simulink model "Standard_H_Infinity_Full_Order_Synthesis"  (R2024a)
settings: Solver=VariableStepAuto  StartTime=0.0  StopTime=10.0  RelTol=1e-3
values from neighbouring files (symbols this model uses):
  Gain_Infinity_Filter_1 = 0.5    [Controller_Stochastic_Optimization.m]    (also in Standard_H_Infinity_Controller_Tuning.m)
  Gain_Infinity_Filter_2 = 100    [Controller_Stochastic_Optimization.m]    (also in Standard_H_Infinity_Controller_Tuning.m = 10000)
  Gain_Infinity_Filter_3 = 10^(Optimal_Vector(5))    [Controller_Stochastic_Optimization.m]    (also in Cost_Function_Optimal_Tuning_Controller.m; Standard_H_Infinity_Controller_Tuning.m = 10)
  Gain_Static_Filter_1 = 1000    [Controller_Stochastic_Optimization.m]    (also in Standard_H_Infinity_Controller_Tuning.m = 100)
  Gain_Static_Filter_2 = 0.01    [Controller_Stochastic_Optimization.m]    (also in Standard_H_Infinity_Controller_Tuning.m)
  Gain_Static_Filter_3 = 10^(Optimal_Vector(4))    [Controller_Stochastic_Optimization.m]    (also in Cost_Function_Optimal_Tuning_Controller.m; Standard_H_Infinity_Controller_Tuning.m = 0.1)
  Gain_Static_Filter_4 = 10^(Optimal_Vector(6))    [Controller_Stochastic_Optimization.m]    (also in Cost_Function_Optimal_Tuning_Controller.m; Standard_H_Infinity_Controller_Tuning.m = 0.1)
  Input_Matrix_Nominal_Global = [Input_Matrix_Nominal Perturbation_Input_Matrix_Nominal]    [Controller_Stochastic_Optimization.m]    (also in Standard_H_Infinity_Controller_Tuning.m)
  Input_Measurement_Matrix_Global_Nominal = [0 0]    [Controller_Stochastic_Optimization.m]    (also in Standard_H_Infinity_Controller_Tuning.m)
  Measurement_Matrix_Ship_Wave_Nominal = [0 1 1 0]    [Controller_Stochastic_Optimization.m]    (also in Standard_H_Infinity_Controller_Tuning.m)
  Pulsation_Unit_Gain_Filter_1 = 10^(Optimal_Vector(1))    [Controller_Stochastic_Optimization.m]    (also in Cost_Function_Optimal_Tuning_Controller.m; Standard_H_Infinity_Controller_Tuning.m = 0.15)
  Pulsation_Unit_Gain_Filter_2 = 10^(Optimal_Vector(2))    [Controller_Stochastic_Optimization.m]    (also in Cost_Function_Optimal_Tuning_Controller.m; Standard_H_Infinity_Controller_Tuning.m = 0.8)
  Pulsation_Unit_Gain_Filter_3 = 10^(Optimal_Vector(3))    [Controller_Stochastic_Optimization.m]    (also in Cost_Function_Optimal_Tuning_Controller.m; Standard_H_Infinity_Controller_Tuning.m = 70)
  State_Matrix_Ship_Wave_Nominal = [0 1 0 0 ... (first row only)    [Controller_Stochastic_Optimization.m]    (also in Standard_H_Infinity_Controller_Tuning.m)
settings Model: Creator=gerar  LastModifiedBy=gerar

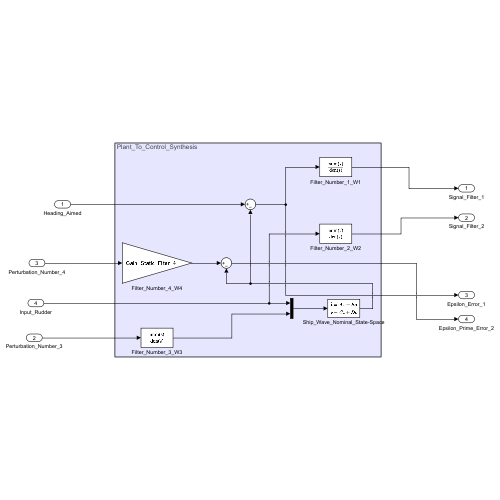
[thumbnail: Simulink's stored preview of the top-level diagram]
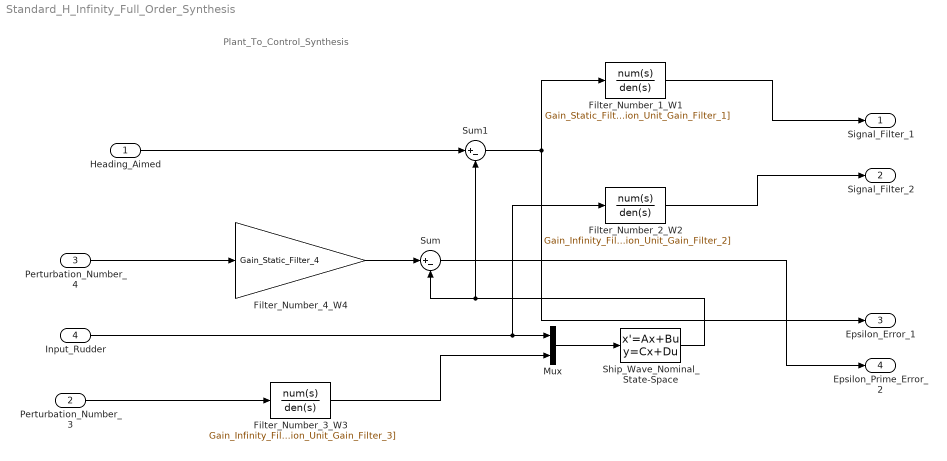
== system Standard_H_Infinity_Full_Order_Synthesis ==
  note: Plant_To_Control_Synthesis
  Heading_Aimed : Inport
  Perturbation_Number_3 : Inport  Port=2
  Perturbation_Number_4 : Inport  Port=3
  Input_Rudder : Inport  Port=4
  Filter_Number_1_W1 : TransferFcn  Numerator=Gain_Static_Filter_1*[Gain_Infinity_Filter_1 Pulsation_Unit_Gain_Filter_1]  Denominator=[Gain_Static_Filter_1 Pulsation_Unit_Gain_Filter_1]
  Filter_Number_2_W2 : TransferFcn  Numerator=Gain_Infinity_Filter_2*[1 Gain_Static_Filter_2*Pulsation_Unit_Gain_Filter_2]  Denominator=[1 Gain_Infinity_Filter_2*Pulsation_Unit_Gain_Filter_2]
  Filter_Number_3_W3 : TransferFcn  Numerator=Gain_Infinity_Filter_3*[1 Gain_Static_Filter_3*Pulsation_Unit_Gain_Filter_3]  Denominator=[1 Gain_Infinity_Filter_3*Pulsation_Unit_Gain_Filter_3]
  Filter_Number_4_W4 : Gain  Gain=Gain_Static_Filter_4
  Mux : Mux  Inputs=2
  Ship_Wave_Nominal_State-Space : StateSpace  A=State_Matrix_Ship_Wave_Nominal  B=Input_Matrix_Nominal_Global  C=Measurement_Matrix_Ship_Wave_Nominal  D=Input_Measurement_Matrix_Global_Nominal  InitialCondition=0
  Sum : Sum  Inputs=|+-
  Sum1 : Sum  Inputs=|+-
  Signal_Filter_1 : Outport
  Signal_Filter_2 : Outport  Port=2
  Epsilon_Error_1 : Outport  Port=3
  Epsilon_Prime_Error_2 : Outport  Port=4
  wires:
  Filter_Number_1_W1/1 -> Signal_Filter_1/1
  Filter_Number_2_W2/1 -> Signal_Filter_2/1
  Sum1/1 -> Epsilon_Error_1/1, Filter_Number_1_W1/1
  Sum/1 -> Epsilon_Prime_Error_2/1
  Heading_Aimed/1 -> Sum1/1
  Perturbation_Number_4/1 -> Filter_Number_4_W4/1
  Perturbation_Number_3/1 -> Filter_Number_3_W3/1
  Filter_Number_4_W4/1 -> Sum/1
  Mux/1 -> Ship_Wave_Nominal_State-Space/1
  Ship_Wave_Nominal_State-Space/1 -> Sum/2, Sum1/2
  Input_Rudder/1 -> Filter_Number_2_W2/1, Mux/1
  Filter_Number_3_W3/1 -> Mux/2
